simulink model "act_4"  (R2025b)
settings: Solver=VariableStepAuto  StartTime=0.0  StopTime=inf  RelTol=1e-3

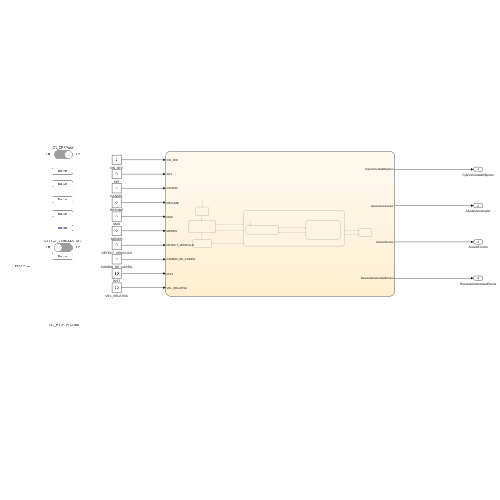
[thumbnail: Simulink's stored preview of the top-level diagram]
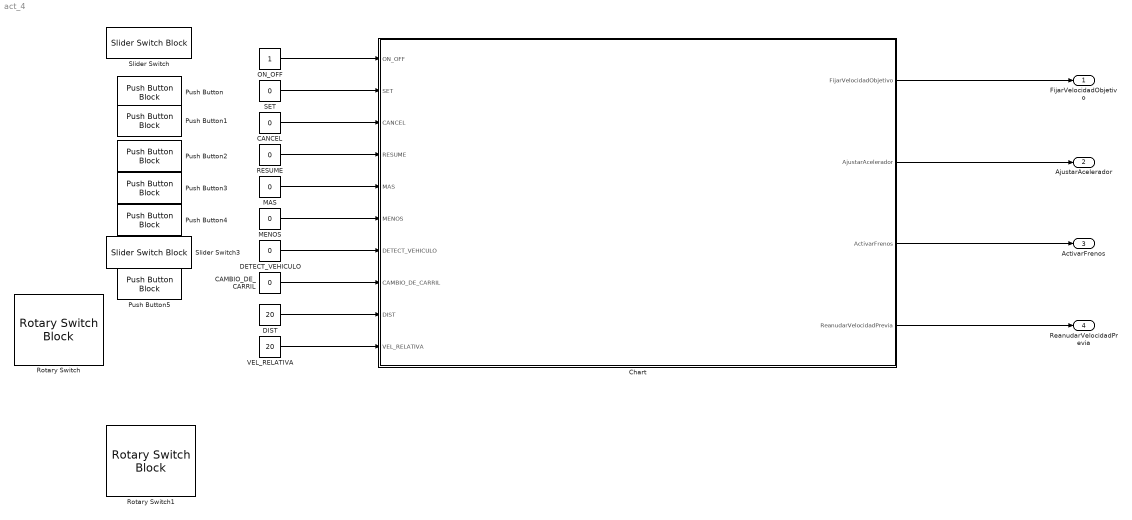
== system act_4 ==
  CAMBIO_DE_CARRIL : Constant  Value=0
  CANCEL : Constant  Value=0
  Chart : Stateflow chart  TreatAsAtomicUnit=on
  DETECT_VEHICULO : Constant  Value=0
  DIST : Constant  Value=20
  MAS : Constant  Value=0
  MENOS : Constant  Value=0
  ON_OFF : Constant
  Push Button{,1..5} (6 alike) : PushButtonBlock  IconOnColor=[0.0, 0.39215686274509803, 0.0]  IconOffColor=[0.0, 1.0, 0.0]  OffValue=0.000000
  RESUME : Constant  Value=0
  Rotary Switch : RotarySwitchBlock
  Rotary Switch1 : RotarySwitchBlock
  SET : Constant  Value=0
  Slider Switch : SliderSwitchBlock
  Slider Switch3 : SliderSwitchBlock
  VEL_RELATIVA : Constant  Value=20
  FijarVelocidadObjetivo : Outport
  AjustarAcelerador : Outport  Port=2
  ActivarFrenos : Outport  Port=3
  ReanudarVelocidadPrevia : Outport  Port=4
  wires:
  ON_OFF/1 -> Chart/1(ON_OFF)
  SET/1 -> Chart/2(SET)
  CANCEL/1 -> Chart/3(CANCEL)
  RESUME/1 -> Chart/4(RESUME)
  MAS/1 -> Chart/5(MAS)
  MENOS/1 -> Chart/6(MENOS)
  DETECT_VEHICULO/1 -> Chart/7(DETECT_VEHICULO)
  CAMBIO_DE_CARRIL/1 -> Chart/8(CAMBIO_DE_CARRIL)
  DIST/1 -> Chart/9(DIST)
  VEL_RELATIVA/1 -> Chart/10(VEL_RELATIVA)
  Chart/1(FijarVelocidadObjetivo) -> FijarVelocidadObjetivo/1
  Chart/2(AjustarAcelerador) -> AjustarAcelerador/1
  Chart/3(ActivarFrenos) -> ActivarFrenos/1
  Chart/4(ReanudarVelocidadPrevia) -> ReanudarVelocidadPrevia/1

== stateflow chart act_4/Chart ==
  state APAGADO
  state ACTIVO
    entry:
    FijarVelocidadObjetivo = 1;
    state SIGUIENDO_OBJETIVO
      during:
      ReanudarVelocidadPrevia = 0;
      if (DIST < 10 && VEL_RELATIVA == 80)
      FijarVelocidadObjetivo = 1;
      end
    state MANTENIENDO_VELOCIDAD
      during:
      ReanudarVelocidadPrevia = 1;
    (default) -> MANTENIENDO_VELOCIDAD
    MANTENIENDO_VELOCIDAD -> SIGUIENDO_OBJETIVO : [DETECT_VEHICULO == 1]
    SIGUIENDO_OBJETIVO -> MANTENIENDO_VELOCIDAD : [CAMBIO_DE_CARRIL == 1]
  state EN_ESPERA
    FijarVelocidadObjetivo = 0;
    AjustarAcelerador = 0;
    ActivarFrenos = 0;
    ReanudarVelocidadPrevia = 0;
  state ANULADO
  state FRENADO_USUARIO
  (default) -> APAGADO
  APAGADO -> EN_ESPERA : [ON_OFF == 1]
  EN_ESPERA -> ACTIVO : [SET == 1 || RESUME ==1]
  ACTIVO -> ANULADO [order 1] : [MAS == 1]
  ACTIVO -> EN_ESPERA [order 3] : [CANCEL ==1]
  FRENADO_USUARIO -> EN_ESPERA : [MENOS == 1]
  ANULADO -> ACTIVO : [MAS == 0]
  ACTIVO -> FRENADO_USUARIO [order 2] : [MENOS == 1]
  data: FijarVelocidadObjetivo output; AjustarAcelerador output; ActivarFrenos output; ON_OFF input; SET input; CANCEL input; RESUME input; MAS input; MENOS input; DETECT_VEHICULO input; CAMBIO_DE_CARRIL input; DIST input; VEL_RELATIVA input; ReanudarVelocidadPrevia output
